simulink model "GalvoModel_v31_dcgain"  (R2013a)
settings: Solver=ode45  StartTime=0.0  StopTime=50e-3  RelTol=1e-3
settings Model: Creator=mainster  LastModifiedBy=mainster

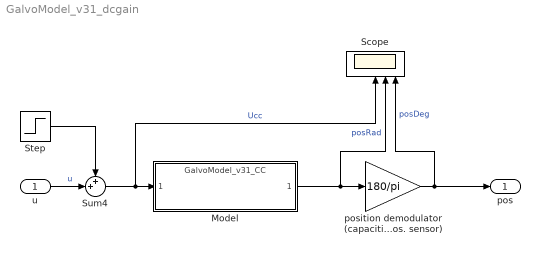
== system GalvoModel_v31_dcgain ==
  u : Inport
  Model : ModelReference  ModelNameDialog=GalvoModel_v31_CC.slx  SimulationMode=Normal  ModelReferenceVersion=1.13  CopyOfModelName=GalvoModel_v31_CC.slx  DefaultDataLogging=on
  Scope : Scope  NumInputPorts=5
      settings: ShowLegends=on  TimeRange=0.05  YMin=-1~-1~0~0~0  YMax=1~1~0.02~0.015~0.8  MaxDataPoints=500000
  Step : Step  Time=1e-3  After=0.02  SampleTime=0
      settings: AttributesFormatString=Ampl.: %<After>
  Sum4 : Sum  Inputs=++|
  position demodulator (capacitive angular pos. sensor) : Gain  Gain=180/pi
  pos : Outport
  wires:
  Sum4/1 -> Scope/3, Model/1  "Ucc"
  Step/1 -> Sum4/1
  u/1 -> Sum4/2  "u"
  Model/1 -> Scope/4, position demodulator (capacitive angular pos. sensor)/1  "posRad"
  position demodulator (capacitive angular pos. sensor)/1 -> pos/1, Scope/5  "posDeg"
